simulink model "BC_ITM_Model"  (R2018a)
settings: Solver=ode4  StartTime=0.0  StopTime=T_end  FixedStep=0.1  RelTol=1e-3
values from neighbouring files (symbols this model uses):
  INV =     [RinehartPM150DZR_ThermalModelParameters.mat]
undefined symbols (not defined in the file or in its folder): COOLANT, DATA
settings Model: Creator=salyer.103  LastModifiedBy=Zach
settings CodeAppCC: StateflowObjectComments=on

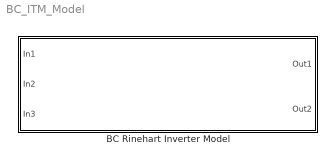
== system BC_ITM_Model ==
  BC Rinehart Inverter Model : Subsystem

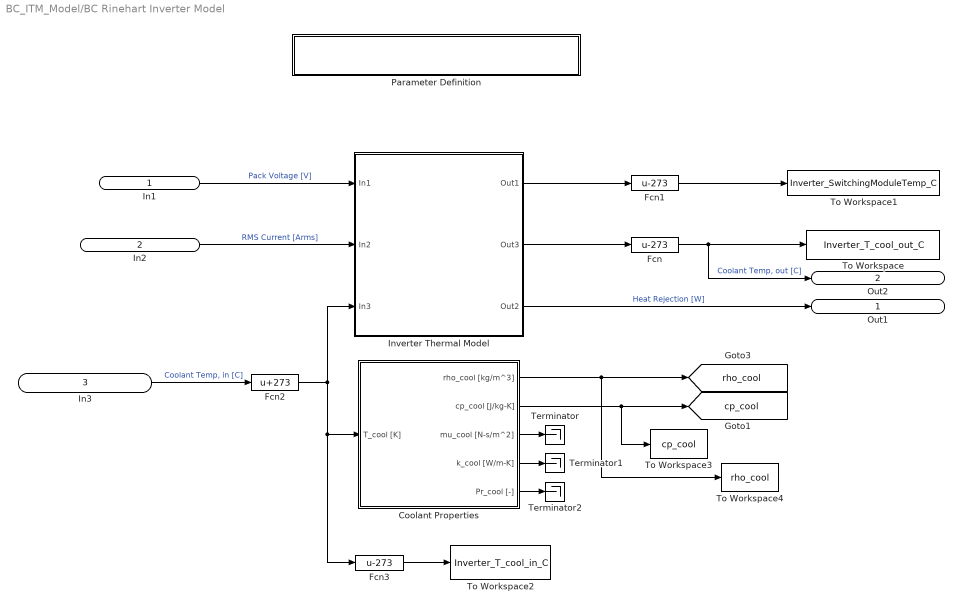
== system BC_ITM_Model/BC Rinehart Inverter Model ==
  In1 : Inport
  In2 : Inport  Port=2
  In3 : Inport  Port=3
  Coolant Properties : Subsystem
  Fcn : Fcn  Expr=u-273
  Fcn1 : Fcn  Expr=u-273
  Fcn2 : Fcn  Expr=u+273
  Fcn3 : Fcn  Expr=u-273
  Inverter Thermal Model : Subsystem
  Parameter Definition : Subsystem
  Terminator : Terminator
  Terminator1 : Terminator
  Terminator2 : Terminator
  To Workspace : ToWorkspace  VariableName=Inverter_T_cool_out_C  SampleTime=-1
  To Workspace1 : ToWorkspace  VariableName=Inverter_SwitchingModuleTemp_C  SampleTime=-1
  To Workspace2 : ToWorkspace  VariableName=Inverter_T_cool_in_C  SampleTime=-1
  To Workspace3 : ToWorkspace  VariableName=cp_cool  SampleTime=-1
  To Workspace4 : ToWorkspace  VariableName=rho_cool  SampleTime=-1
  Out1 : Outport
  Out2 : Outport  Port=2
  tag scope: cp_cool=global, rho_cool=global
  wires:
  In1/1 -> Inverter Thermal Model/1(In1)  "Pack Voltage [V]"
  Fcn1/1 -> To Workspace1/1
  Coolant Properties/2(cp_cool [J/kg-K]) -> To Workspace3/1, [cp_cool]
  Fcn/1 -> Out2/1, To Workspace/1  "Coolant Temp, out [C]"
  Coolant Properties/1(rho_cool [kg/m^3]) -> To Workspace4/1, [rho_cool]
  Inverter Thermal Model/1(Out1) -> Fcn1/1
  Coolant Properties/3(mu_cool [N-s/m^2]) -> Terminator/1
  Fcn2/1 -> Inverter Thermal Model/3(In3), Fcn3/1, Coolant Properties/1(T_cool [K])
  Fcn3/1 -> To Workspace2/1
  Coolant Properties/5(Pr_cool [-]) -> Terminator2/1
  Coolant Properties/4(k_cool [W/m-K]) -> Terminator1/1
  Inverter Thermal Model/2(Out3) -> Fcn/1
  In2/1 -> Inverter Thermal Model/2(In2)  "RMS Current [Arms]"
  In3/1 -> Fcn2/1  "Coolant Temp, in [C]"
  Inverter Thermal Model/3(Out2) -> Out1/1  "Heat Rejection [W]"

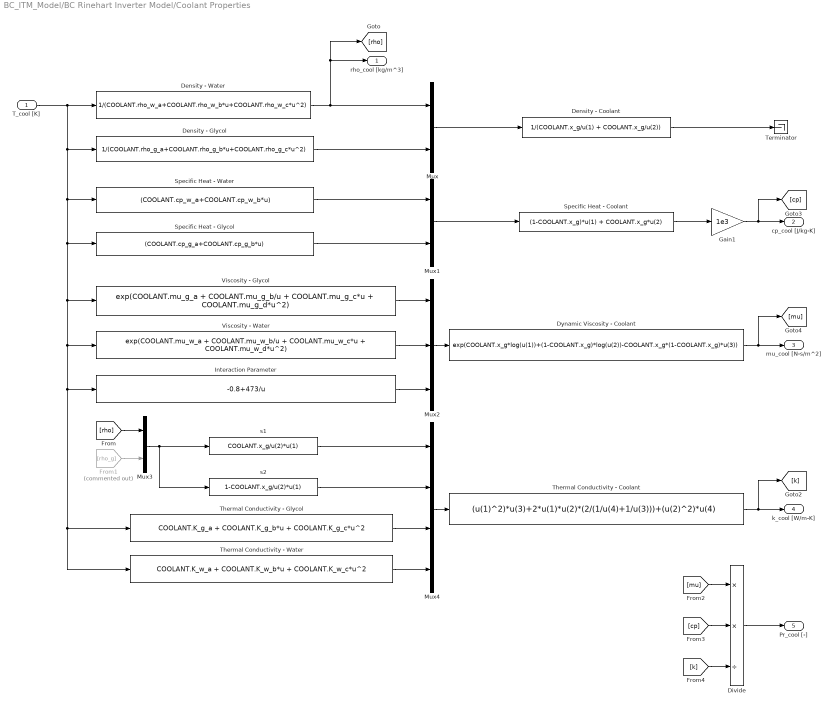
== system BC_ITM_Model/BC Rinehart Inverter Model/Coolant Properties ==
  T_cool [K] : Inport
  Density - Coolant : Fcn  Expr=1/(COOLANT.x_g/u(1) + COOLANT.x_g/u(2))
  Density - Glycol : Fcn  Expr=1/(COOLANT.rho_g_a+COOLANT.rho_g_b*u+COOLANT.rho_g_c*u^2)
  Density - Water : Fcn  Expr=1/(COOLANT.rho_w_a+COOLANT.rho_w_b*u+COOLANT.rho_w_c*u^2)
  Divide : Product  Inputs=**/
  Dynamic Viscosity - Coolant : Fcn  Expr=exp(COOLANT.x_g*log(u(1))+(1-COOLANT.x_g)*log(u(2))-COOLANT.x_g*(1-COOLANT.x_g)*u(3))
  From1 : From  Commented=on  GotoTag=rho_g
  Gain1 : Gain  Gain=1e3
  Interaction Parameter : Fcn  Expr=-0.8+473/u
  Mux : Mux  Inputs=2
  Mux1 : Mux  Inputs=2
  Mux2 : Mux  Inputs=3
  Mux3 : Mux  Inputs=2
  Mux4 : Mux
  Specific Heat - Coolant : Fcn  Expr=(1-COOLANT.x_g)*u(1) + COOLANT.x_g*u(2)
  Specific Heat - Glycol : Fcn  Expr=(COOLANT.cp_g_a+COOLANT.cp_g_b*u)
  Specific Heat - Water : Fcn  Expr=(COOLANT.cp_w_a+COOLANT.cp_w_b*u)
  Terminator : Terminator
  Thermal Conductivity - Coolant : Fcn  Expr=(u(1)^2)*u(3)+2*u(1)*u(2)*(2/(1/u(4)+1/u(3)))+(u(2)^2)*u(4)
  Thermal Conductivity - Glycol : Fcn  Expr=COOLANT.K_g_a + COOLANT.K_g_b*u + COOLANT.K_g_c*u^2
  Thermal Conductivity - Water : Fcn  Expr=COOLANT.K_w_a + COOLANT.K_w_b*u + COOLANT.K_w_c*u^2
  Viscosity - Glycol : Fcn  Expr=exp(COOLANT.mu_g_a + COOLANT.mu_g_b/u + COOLANT.mu_g_c*u + COOLANT.mu_g_d*u^2)
  Viscosity - Water : Fcn  Expr=exp(COOLANT.mu_w_a + COOLANT.mu_w_b/u + COOLANT.mu_w_c*u + COOLANT.mu_w_d*u^2)
  s1 : Fcn  Expr=COOLANT.x_g/u(2)*u(1)
  s2 : Fcn  Expr=1-COOLANT.x_g/u(2)*u(1)
  rho_cool [kg/m^3] : Outport
  cp_cool [J/kg-K] : Outport  Port=2
  mu_cool [N-s/m^2] : Outport  Port=3
  k_cool [W/m-K] : Outport  Port=4
  Pr_cool [-] : Outport  Port=5
  wires:
  Density - Coolant/1 -> Terminator/1
  Mux/1 -> Density - Coolant/1
  T_cool [K]/1 -> Density - Water/1, Density - Glycol/1, Specific Heat - Water/1, Specific Heat - Glycol/1, Viscosity - Glycol/1, Viscosity - Water/1, Interaction Parameter/1, Thermal Conductivity - Glycol/1, Thermal Conductivity - Water/1
  Specific Heat - Coolant/1 -> Gain1/1
  Gain1/1 -> cp_cool [J/kg-K]/1, [cp]
  Mux2/1 -> Dynamic Viscosity - Coolant/1
  Viscosity - Glycol/1 -> Mux2/1
  Viscosity - Water/1 -> Mux2/2
  Interaction Parameter/1 -> Mux2/3
  Density - Water/1 -> Mux/1, rho_cool [kg/m^3]/1, [rho]
  Density - Glycol/1 -> Mux/2
  Dynamic Viscosity - Coolant/1 -> mu_cool [N-s/m^2]/1, [mu]
  Specific Heat - Water/1 -> Mux1/1
  Specific Heat - Glycol/1 -> Mux1/2
  Mux1/1 -> Specific Heat - Coolant/1
  Thermal Conductivity - Glycol/1 -> Mux4/3
  Thermal Conductivity - Water/1 -> Mux4/4
  Mux4/1 -> Thermal Conductivity - Coolant/1
  [rho] -> Mux3/1
  From1/1 -> Mux3/2
  Mux3/1 -> s1/1, s2/1
  s1/1 -> Mux4/1
  s2/1 -> Mux4/2
  Thermal Conductivity - Coolant/1 -> k_cool [W/m-K]/1, [k]
  Divide/1 -> Pr_cool [-]/1
  [mu] -> Divide/1
  [cp] -> Divide/2
  [k] -> Divide/3

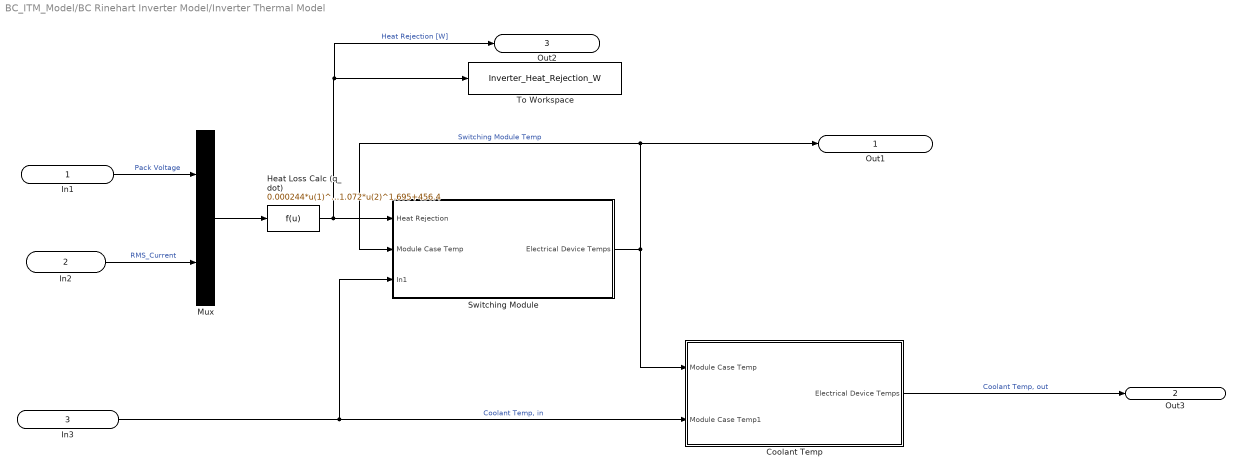
== system BC_ITM_Model/BC Rinehart Inverter Model/Inverter Thermal Model ==
  In1 : Inport
  In2 : Inport  Port=2
  In3 : Inport  Port=3
  Coolant Temp : Subsystem
  Heat Loss Calc (q_dot) : Fcn  Expr=0.000244*u(1)^1.072*u(2)^1.695+456.4
  Mux : Mux  Inputs=2
  Switching Module : Subsystem
  To Workspace : ToWorkspace  VariableName=Inverter_Heat_Rejection_W  SampleTime=-1
  Out1 : Outport
  Out3 : Outport  Port=2
  Out2 : Outport  Port=3
  wires:
  In1/1 -> Mux/1  "Pack Voltage"
  In2/1 -> Mux/2  "RMS_Current"
  Mux/1 -> Heat Loss Calc (q_dot)/1
  Heat Loss Calc (q_dot)/1 -> Out2/1, To Workspace/1, Switching Module/1(Heat Rejection)  "Heat Rejection [W]"
  Switching Module/1(Electrical Device Temps) -> Coolant Temp/1(Module Case Temp), Out1/1, Switching Module/2(Module Case Temp)  "Switching Module Temp"
  In3/1 -> Switching Module/3(In1), Coolant Temp/2(Module Case Temp1)  "Coolant Temp, in"
  Coolant Temp/1(Electrical Device Temps) -> Out3/1  "Coolant Temp, out"

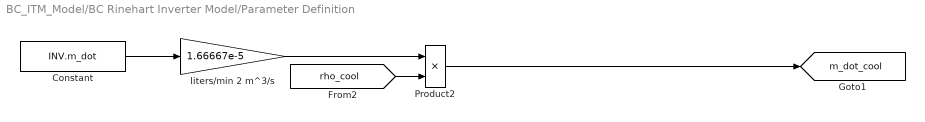
== system BC_ITM_Model/BC Rinehart Inverter Model/Parameter Definition ==
  Constant : Constant  Value=INV.m_dot
  Product2 : Product
  liters/min 2 m^3/s : Gain  Gain=1.66667e-5
  tag scope: m_dot_cool=global
  wires:
  Constant/1 -> liters/min 2 m^3/s/1
  Product2/1 -> [m_dot_cool]
  [rho_cool] -> Product2/2
  liters/min 2 m^3/s/1 -> Product2/1

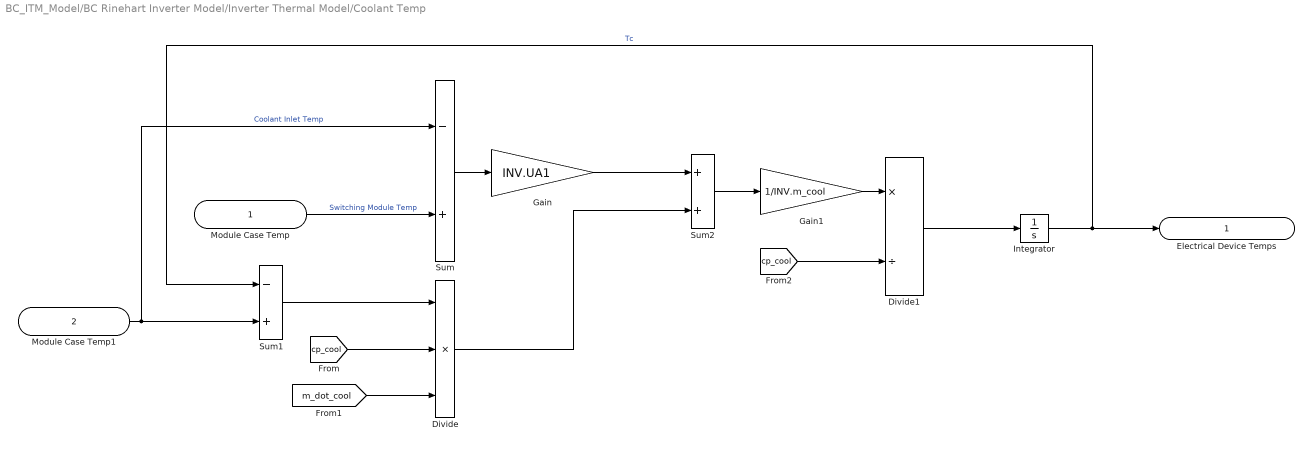
== system BC_ITM_Model/BC Rinehart Inverter Model/Inverter Thermal Model/Coolant Temp ==
  Module Case Temp : Inport
  Module Case Temp1 : Inport  Port=2
  Divide : Product  Inputs=***
  Divide1 : Product  Inputs=*/
  Gain : Gain  Gain=INV.UA1
  Gain1 : Gain  Gain=1/INV.m_cool
  Integrator : Integrator  InitialCondition=DATA.ITM(1,2)+273
  Sum : Sum  Inputs=-+
  Sum1 : Sum  Inputs=-+
  Sum2 : Sum
  Electrical Device Temps : Outport
  wires:
  Module Case Temp/1 -> Sum/2  "Switching Module Temp"
  Sum/1 -> Gain/1
  Gain/1 -> Sum2/1
  Divide/1 -> Sum2/2
  [cp_cool] -> Divide/2
  [m_dot_cool] -> Divide/3
  Gain1/1 -> Divide1/1
  Integrator/1 -> Sum1/1, Electrical Device Temps/1  "Tc"
  [cp_cool] -> Divide1/2
  Divide1/1 -> Integrator/1
  Sum2/1 -> Gain1/1
  Module Case Temp1/1 -> Sum/1, Sum1/2  "Coolant Inlet Temp"
  Sum1/1 -> Divide/1

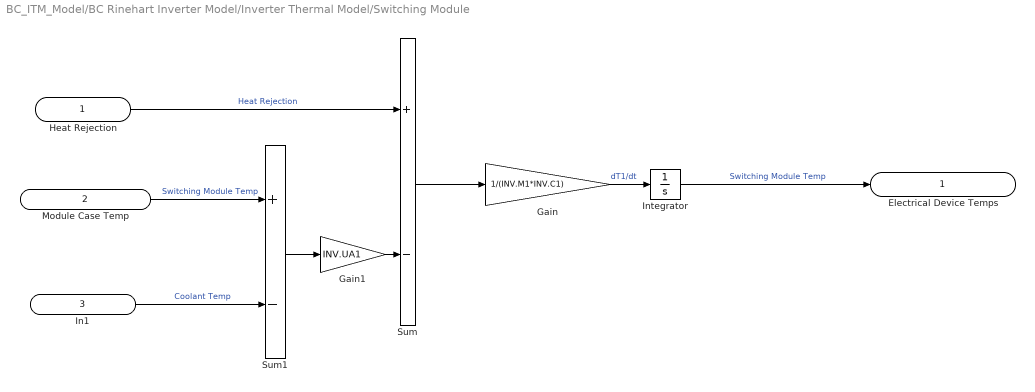
== system BC_ITM_Model/BC Rinehart Inverter Model/Inverter Thermal Model/Switching Module ==
  Heat Rejection : Inport
  Module Case Temp : Inport  Port=2
  In1 : Inport  Port=3
  Gain : Gain  Gain=1/(INV.M1*INV.C1)
  Gain1 : Gain  Gain=INV.UA1
  Integrator : Integrator  InitialCondition=INV.T_init
  Sum : Sum  Inputs=+-
  Sum1 : Sum  Inputs=+-
  Electrical Device Temps : Outport
  wires:
  Heat Rejection/1 -> Sum/1  "Heat Rejection"
  Module Case Temp/1 -> Sum1/1  "Switching Module Temp"
  Integrator/1 -> Electrical Device Temps/1  "Switching Module Temp"
  In1/1 -> Sum1/2  "Coolant Temp"
  Sum/1 -> Gain/1
  Sum1/1 -> Gain1/1
  Gain1/1 -> Sum/2
  Gain/1 -> Integrator/1  "dT1/dt"
